simulink model "dspdltmd"  (Simulink 5.0)
settings: Solver=FixedStepDiscrete  SolverMode=SingleTasking  StartTime=0.0  StopTime=1  RelTol=1e-3
libraries: dspwvfmcdlib x6, dspsrcs4 x1
settings Model: CovMetricSettings=d  Creator=sconahan  LastModifiedBy=mkhan  SaveTime=off  SaveOutput=off  LimitDataPoints=off  RTWOptions="-aExtMode=0 -aForceParamTrailComments=0 -aInlineInvariantSignals=0 -aLocalBlockOutputs=1 -aLogVarNameModifier=\"rt_\" -aRTWVerbose=1 -aRollThreshold=5 -aShowEliminatedStatements=1"  ExtModeTrigMode=oneshot  ExtModeArmWhenConnect=off  BlockReductionOpt=off  BooleanDataType=off

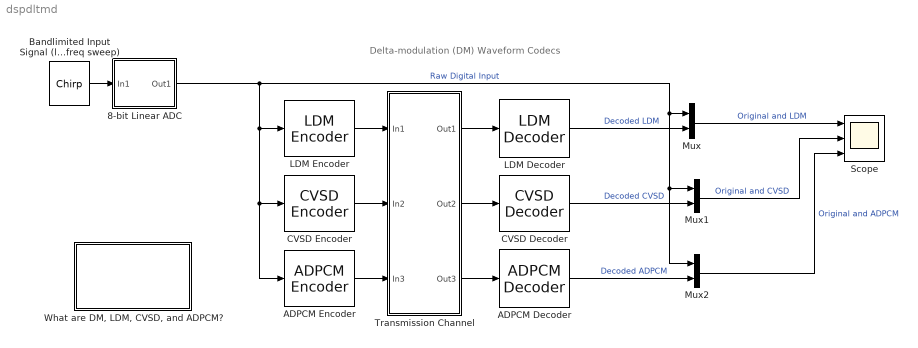
== system dspdltmd ==
  note: Delta-modulation (DM) Waveform Codecs
  8-bit Linear ADC : Subsystem
      settings: RTWFcnNameOpts=Auto  RTWFileNameOpts=Auto
      mask Display: disp('8-bit\nLinear\nQuantizer')
  ADPCM Decoder : dspwvfmcdlib/ADPCM Decoder  StepAttn=.5  StepGain=2  StepMax=0.5  StepMin=0.01  StepInit=0.1  AdpcmIntTau=0.99
  ADPCM Encoder : dspwvfmcdlib/ADPCM Encoder  EncStepAttn=.5  EncStepGain=2  EncStepMax=0.5  EncStepMin=0.01  EncStepInit=0.1  EncIntTau=0.99
  Bandlimited Input Signal (linear freq sweep) : dspsrcs4/Chirp  sweep=Linear  mode=Unidirectional  f0=0  f1=4000  t1=1  Tsweep=1  phase=0  Ts=1/16000  spf=1  datatype=Double
  CVSD Decoder : dspwvfmcdlib/CVSD Decoder  DeltaMax=20  SylIntTau=0.99  DeltaMin=0.01  RecIntTau=0.96
  CVSD Encoder : dspwvfmcdlib/CVSD Encoder  EncDeltaMax=20  EncSylIntTau=0.99  EncDeltaMin=0.01  EncRecIntTau=0.96
  LDM Decoder : dspwvfmcdlib/LDM Decoder  Tau=0.91
  LDM Encoder : dspwvfmcdlib/LDM Encoder  EncTau=0.91
  Mux : Mux  Inputs=2
  Mux1 : Mux  Inputs=2
  Mux2 : Mux  Inputs=2
  Scope : Scope  NumInputPorts=3
      settings: TickLabels=on  TimeRange=1  YMin=-1~-2~-2  YMax=1~2~2  SaveToWorkspace=off  SaveName=ScopeData  LimitDataPoints=on  MaxDataPoints=500000
  Transmission Channel : Subsystem
      settings: RTWFcnNameOpts=Auto  RTWFileNameOpts=Auto
  "What are DM, LDM, CVSD, and ADPCM?" : Subsystem
      settings: RTWFcnNameOpts=Auto  RTWFileNameOpts=Auto
      mask Type: Delta-modulation Demo Info
      mask Display: disp('What are DM,\nLDM, CVSD,\nand ADPCM?')
  wires:
  CVSD Decoder/1 -> Mux1/2  "Decoded CVSD"
  LDM Decoder/1 -> Mux/2  "Decoded LDM"
  LDM Encoder/1 -> Transmission Channel/1(In1)
  CVSD Encoder/1 -> Transmission Channel/2(In2)
  Bandlimited Input Signal (linear freq sweep)/1 -> 8-bit Linear ADC/1(In1)
  8-bit Linear ADC/1(Out1) -> Mux/1, Mux1/1, Mux2/1, LDM Encoder/1, ADPCM Encoder/1, CVSD Encoder/1  "Raw Digital Input"
  Transmission Channel/1(Out1) -> LDM Decoder/1
  Mux/1 -> Scope/1  "Original and LDM"
  ADPCM Encoder/1 -> Transmission Channel/3(In3)
  ADPCM Decoder/1 -> Mux2/2  "Decoded ADPCM"
  Transmission Channel/2(Out2) -> CVSD Decoder/1
  Mux1/1 -> Scope/2  "Original and CVSD"
  Mux2/1 -> Scope/3  "Original and ADPCM"
  Transmission Channel/3(Out3) -> ADPCM Decoder/1

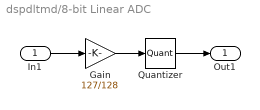
== system dspdltmd/8-bit Linear ADC ==
  In1 : Inport  Port=1  LatchInput=off
  Gain : Gain  Gain=127/128  Multiplication=Element-wise(K.*u)  SaturateOnIntegerOverflow=on
  Quantizer : Quantizer  QuantizationInterval=1/128  LinearizeAsGain=off
  Out1 : Outport  Port=1
  wires:
  Gain/1 -> Quantizer/1
  In1/1 -> Gain/1
  Quantizer/1 -> Out1/1

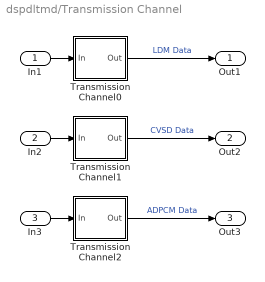
== system dspdltmd/Transmission Channel ==
  In1 : Inport  Port=1  LatchInput=off
  In2 : Inport  Port=2  LatchInput=off
  In3 : Inport  Port=3  LatchInput=off
  Transmission Channel0 : Subsystem
      settings: RTWFcnNameOpts=Auto  RTWFileNameOpts=Auto
  Transmission Channel1 : Subsystem
      settings: RTWFcnNameOpts=Auto  RTWFileNameOpts=Auto
  Transmission Channel2 : Subsystem
      settings: RTWFcnNameOpts=Auto  RTWFileNameOpts=Auto
  Out1 : Outport  Port=1
  Out2 : Outport  Port=2
  Out3 : Outport  Port=3
  wires:
  Transmission Channel0/1(Out) -> Out1/1  "LDM Data"
  In1/1 -> Transmission Channel0/1(In)
  Transmission Channel1/1(Out) -> Out2/1  "CVSD Data"
  In2/1 -> Transmission Channel1/1(In)
  Transmission Channel2/1(Out) -> Out3/1  "ADPCM Data"
  In3/1 -> Transmission Channel2/1(In)

== system dspdltmd/What are DM, LDM, CVSD, and ADPCM? ==
  note: What are DM, LDM, CVSD, and ADPCM?
      |
      | Delta-modulation (DM) is a differential waveform quantization
      | (or coding) technique.  A DM encoder uses the error between
      | the original signal to be coded and the coded signal itself to create
      | a differentially-quantized data stream.  This data stream (usually
      | the computed error signal) is a lower-bit-rate signal that can be
      | decoded by a matched decoder on the receiver side in order to
      | achieve data compression and hence low data transmission rates.
      |
      | Linear Delta-modulation (LDM), Continuously Variable Slope
      | Delta-modulation (CVSD), and Adaptive Differential Pulse Code Modulation
      | (ADPCM) are each differential waveform coding techniques.  Each employ
      | two-level (i.e. one-bit) encoders, and may be performed at many different
      | sampling/data rates.  The encoded bit rate is usually directly proportional
      | to the input signal sample rate.  For example, in both LDM and CVSD
      | one-bit per sample is used to compute the encoded data stream.
      |
      | In LDM, a constant step-size is used to approximate the input signal with
      | a single-bit per signal sample.  In the encoded bit-stream, each "1" bit
      | means "increase the amplitude" by the step-size (as compared to the
      | previous decoded signal sample), while a "0" bit means "decrease the
      | amplitude" by the step-size (as compared to the previous decoded
      | signal sample).  Using LDM, the encoder performance can suffer due to
      | a condition known as "slope-overload", when the input signal slope
      | (such as during high frequency content) changes too rapidly for the
      | encoder to track it accurately.
      |
      | CVSD is basically LDM with the addition of an adaptive step-size.
      | By adjusting (adapting) the step-size to the changes in slope of the
      | input signal, the encoder is able to represent low-frequency signals
      | with greater accuracy without sacrificing as much performance due
      | to "slope-overload" at higher frequencies.  When the slope of the
      | input signal changes too quickly for the encoder to keep up with it,
      | the step-size is increased.  Conversely, when the input signal slope
      | changes slowly, the step-size is decreased.  A slope-overload detector
      | and syllabic filter is used in conjunction with a pulse amplitude
      | modulator (PAM) to accomplish the step-size adaptation.
      |
      | CVSD is used in both commerical and military communications where
      | "toll quality" or "communications quality" is required, yet low computation
      | complexity and low memory requirements are desirable.  Two examples
      | of this technique are U.S. MIL-STD-188-113 (16 kbs and 32kbs CVSD)
      | and U.S. Federal Standard 1023 (12 kbs CVSD).  In addition, encoded
      | CVSD data can be encrypted and made more secure - desirable for
      | many wireless communications applications (including speech
      | and general-purpose audio coding).
      |
      | ADPCM is a lot like CVSD, however it provides more accuracy (and thus
      | preserved frequency bandwidth) at the expense of additional computational
      | requirements for the adaptation step-size calculations.

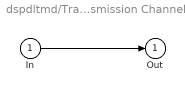
== system dspdltmd/Transmission Channel/Transmission Channel0 ==
  In : Inport  Port=1  LatchInput=off
  Out : Outport  Port=1  InitialOutput=0
  wires:
  In/1 -> Out/1

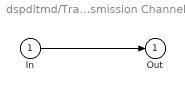
== system dspdltmd/Transmission Channel/Transmission Channel1 ==
  In : Inport  Port=1  LatchInput=off
  Out : Outport  Port=1  InitialOutput=0
  wires:
  In/1 -> Out/1

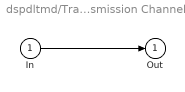
== system dspdltmd/Transmission Channel/Transmission Channel2 ==
  In : Inport  Port=1  LatchInput=off
  Out : Outport  Port=1  InitialOutput=0
  wires:
  In/1 -> Out/1
